simulink subsystem "MPU_SubSystem"  (R2020b)
settings: Solver=VariableStepAuto  StartTime=0.0  StopTime=10.0  RelTol=1e-3
settings Model: Creator=umberto  LastModifiedBy=umberto

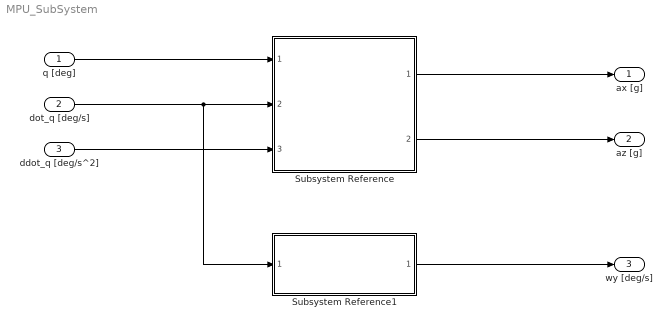
== system MPU_SubSystem ==
  q [deg] : Inport
  dot_q [deg/s] : Inport  Port=2
  ddot_q [deg/s^2] : Inport  Port=3
  Subsystem Reference : Subsystem  ReferencedSubsystem=Accelerometer_SubSystem
  Subsystem Reference1 : Subsystem  ReferencedSubsystem=Gyroscope_SubSystem
  ax [g] : Outport
  az [g] : Outport  Port=2
  wy [deg/s] : Outport  Port=3
  wires:
  Subsystem Reference1/1 -> wy [deg/s]/1
  Subsystem Reference/2 -> az [g]/1
  Subsystem Reference/1 -> ax [g]/1
  ddot_q [deg/s^2]/1 -> Subsystem Reference/3
  dot_q [deg/s]/1 -> Subsystem Reference/2, Subsystem Reference1/1
  q [deg]/1 -> Subsystem Reference/1
